simulink model "mod2_2bit_NO_DEM"  (Simulink 7.9)
settings: Solver=ode45  StartTime=0.0  StopTime=simu.trantime  RelTol=1e-3
undefined symbols (not defined in the file): dac, Fs, mod, OSR, sinamp, sinfreq
libraries: simulink x4, dspsigops x3, dsparch4 x1, dspsrcs4 x1
settings Model: Creator=amyles  LastModifiedBy=Arnaldi Isacco
settings DataIOCC: MaxDataPoints=50000  SaveOutput=off  SaveTime=off
settings DebuggingCC: ParameterPrecisionLossMsg=none  StrictBusMsg=Warning
settings SFSimCC: SimParseCustomCode=off
settings CodeAppCC: CustomSymbolStrType=$N$R$M_T
settings GRTTargetCC: CombineOutputUpdateFcns=off  GRTInterface=on

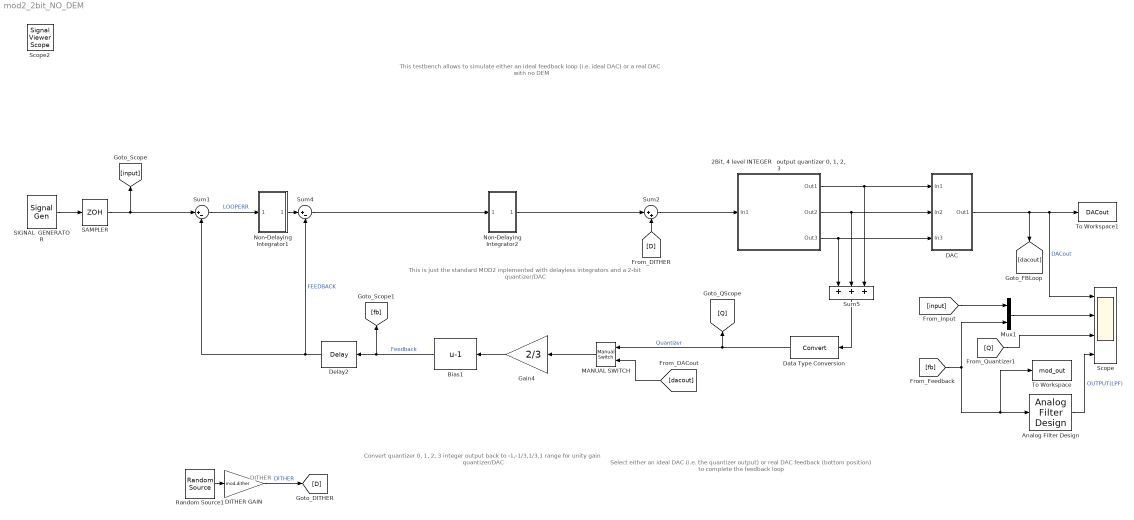
== system mod2_2bit_NO_DEM ==
  note: Convert quantizer 0, 1, 2, 3 integer
      | output back  to -1,-1/3,1/3,1 range for
      | unity gain quantizer/DAC
  note: Select either an ideal DAC
      | (i.e. the quantizer output) or real
      | DAC feedback (bottom position) to
      | complete the feedback loop
  note: This testbench allows to simulate either an ideal feedback loop (i.e. ideal DAC) or a real DAC with no DEM
  note: This is just the standard MOD2 inplemented with delayless integrators and a 2-bit quantizer/DAC
  note: DITHER
  "2Bit, 4 level INTEGER   output quantizer 0, 1, 2, 3" : Subsystem
  Analog Filter Design : dsparch4/Analog Filter Design  method=Butterworth  filttype=Lowpass  N=8  Wlo=pi*(Fs/OSR)  Whi=80  Rp=2  Rs=40
      settings: AttributesFormatString=Low-pass filter the loop output\nto illustrate intuitively how the\npulse density modulated +1/-1\noutput stream does indeed capture\nthe input signal
  Bias1 : Bias  Bias=-1
  DAC : Subsystem
  DITHER GAIN : Gain  Gain=mod.dither  SampleTime=1/Fs
  Data Type Conversion : DataTypeConversion
  Delay2 : dspsigops/Delay  InputProcessing=Columns as channels (frame based)  dly_unit=Samples  delay=1  ic_detail=off  dif_ic_for_ch=off  dif_ic_for_dly=off  ic=0  reset_popup=None
  Gain4 : Gain  Gain=2/3  SampleTime=1/Fs
  MANUAL SWITCH : simulink/Signal Routing/Manual Switch  sw=0  action=0  varsize=off
      settings: AttributesFormatString=Double click to\nselect the desired\ninput
  Mux1 : Mux  Inputs=2
  Non-Delaying Integrator1 : Subsystem
  Non-Delaying Integrator2 : Subsystem
  Random Source1 : dspsrcs4/Random Source  SrcType=Uniform  NormMethod=Ziggurat  CltLength=12  MinVal=-1  MaxVal=1  MeanVal=0  VarVal=1  RepMode=Not repeatable  rawSeed=1  IsInherit=off  SampMode=Discrete  SampTime=1/Fs  SampFrame=1  DataType=Double  OutComplex=Real
  SAMPLER : ZeroOrderHold  SampleTime=1/Fs
  SIGNAL  GENERATOR : SignalGenerator  Amplitude=sinamp  Frequency=sinfreq  VectorParams1D=off
  Scope : Scope  NumInputPorts=4
      settings: YMin=-0.2~-1.1~-0.2~-1.1  YMax=3.2~1.1~3.2~1.1
  Sum1 : Sum  Inputs=|+-  SampleTime=1/Fs
      settings: AttributesFormatString=Modulator input\nloop servo error (input - fbk)
  Sum2 : Sum  Inputs=|++
  Sum4 : Sum  Inputs=|+-
  Sum5 : Sum  Inputs=+++  SampleTime=1/Fs
  To Workspace : ToWorkspace  VariableName=mod_out  SampleTime=-1
  To Workspace1 : ToWorkspace  VariableName=DACout  SampleTime=-1
  Scope2 : SignalViewerScope  IOType=viewer  NumInputPorts=5  ZoomMode=yonly  RefreshTime=0.035000
      settings: YMin=-5~-5~-5~-5~-5  YMax=5~5~5~5~5
  wires:
  Sum1/1 -> Non-Delaying Integrator1/1(In1)  "LOOPERR"
  Delay2/1 -> Sum1/2, Sum4/2  "FEEDBACK"
  SAMPLER/1 -> Sum1/1, [input]
  Sum4/1 -> Non-Delaying Integrator2/1(In1)
  [D] -> Sum2/2
  MANUAL SWITCH/1 -> Gain4/1
  Bias1/1 -> Delay2/1, [fb]  "Feedback"
  Gain4/1 -> Bias1/1
  Sum2/1 -> "2Bit, 4 level INTEGER   output quantizer 0, 1, 2, 3"/1(In1)
  Non-Delaying Integrator1/1(Out1) -> Sum4/1
  Non-Delaying Integrator2/1(Out1) -> Sum2/1
  Data Type Conversion/1 -> MANUAL SWITCH/1, [Q]  "Quantizer"
  [dacout] -> MANUAL SWITCH/2
  "2Bit, 4 level INTEGER   output quantizer 0, 1, 2, 3"/3(Out3) -> Sum5/1, DAC/3(In3)
  "2Bit, 4 level INTEGER   output quantizer 0, 1, 2, 3"/2(Out2) -> Sum5/2, DAC/2(In2)
  Sum5/1 -> Data Type Conversion/1
  "2Bit, 4 level INTEGER   output quantizer 0, 1, 2, 3"/1(Out1) -> Sum5/3, DAC/1(In1)
  DAC/1(Out1) -> [dacout], To Workspace1/1, Scope/1  "DACout"
  [input] -> Mux1/1
  Random Source1/1 -> DITHER GAIN/1
  DITHER GAIN/1 -> [D]  "DITHER"
  SIGNAL  GENERATOR/1 -> SAMPLER/1
  [fb] -> Mux1/2, Analog Filter Design/1, To Workspace/1
  Mux1/1 -> Scope/2
  [Q] -> Scope/3
  Analog Filter Design/1 -> Scope/4  "OUTPUT(LPF)"

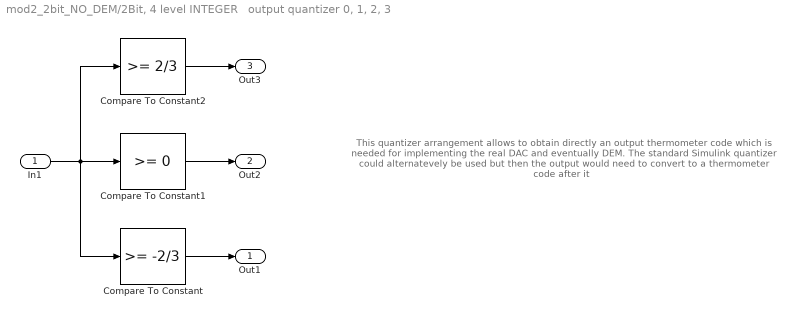
== system mod2_2bit_NO_DEM/2Bit, 4 level INTEGER   output quantizer 0, 1, 2, 3 ==
  note: This quantizer arrangement allows to obtain directly
      | an output thermometer code which is needed for implementing
      | the real DAC and eventually DEM. The standard Simulink
      | quantizer could alternatevely be used but then the output
      | would need to convert to a thermometer code after it
  In1 : Inport
  Compare To Constant : simulink/Logic and Bit Operations/Compare To Constant  relop=>=  const=-2/3  OutDataTypeStr=uint8
  Compare To Constant1 : simulink/Logic and Bit Operations/Compare To Constant  relop=>=  const=0  OutDataTypeStr=uint8
  Compare To Constant2 : simulink/Logic and Bit Operations/Compare To Constant  relop=>=  const=2/3  OutDataTypeStr=uint8
  Out1 : Outport
  Out2 : Outport  Port=2
  Out3 : Outport  Port=3
  wires:
  In1/1 -> Compare To Constant/1, Compare To Constant1/1, Compare To Constant2/1
  Compare To Constant/1 -> Out1/1
  Compare To Constant1/1 -> Out2/1
  Compare To Constant2/1 -> Out3/1

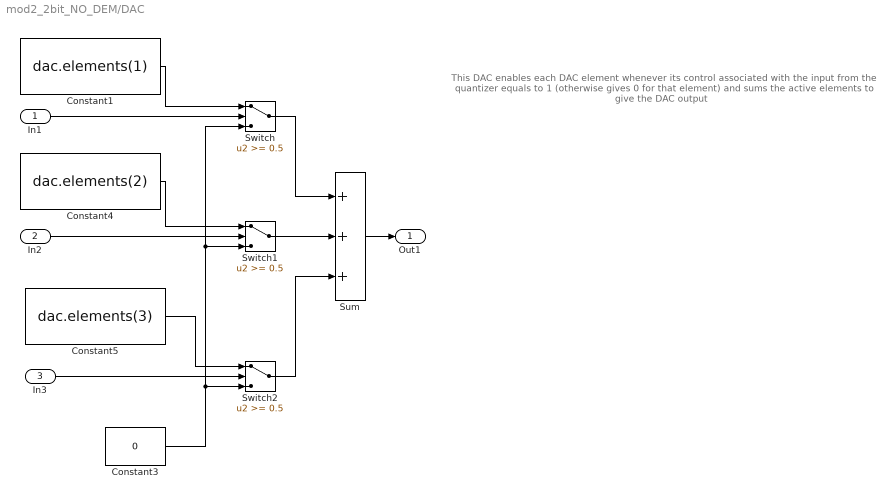
== system mod2_2bit_NO_DEM/DAC ==
  note: This DAC enables each DAC element whenever its control associated
      | with the input from the quantizer equals to 1 (otherwise gives 0 for that
      | element) and sums the active elements to give the DAC output
  In1 : Inport
  In2 : Inport  Port=2
  In3 : Inport  Port=3
  Constant1 : Constant  Value=dac.elements(1)  SampleTime=1/Fs
  Constant3 : Constant  Value=0  SampleTime=1/Fs
  Constant4 : Constant  Value=dac.elements(2)  SampleTime=1/Fs
  Constant5 : Constant  Value=dac.elements(3)  SampleTime=1/Fs
  Sum : Sum  Inputs=+++
  Switch : Switch  Threshold=0.5  SampleTime=1/Fs
  Switch1 : Switch  Threshold=0.5  SampleTime=1/Fs
  Switch2 : Switch  Threshold=0.5  SampleTime=1/Fs
  Out1 : Outport
  wires:
  Switch/1 -> Sum/1
  Switch1/1 -> Sum/2
  Switch2/1 -> Sum/3
  Sum/1 -> Out1/1
  In1/1 -> Switch/2
  In2/1 -> Switch1/2
  In3/1 -> Switch2/2
  Constant1/1 -> Switch/1
  Constant3/1 -> Switch2/3, Switch1/3, Switch/3
  Constant4/1 -> Switch1/1
  Constant5/1 -> Switch2/1

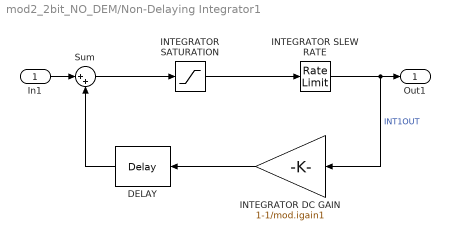
== system mod2_2bit_NO_DEM/Non-Delaying Integrator1 ==
  In1 : Inport
  DELAY : dspsigops/Delay  InputProcessing=Inherited (this choice will be removed - see release notes)  dly_unit=Samples  delay=1  ic_detail=off  dif_ic_for_ch=off  dif_ic_for_dly=off  ic=0  reset_popup=None
  INTEGRATOR SATURATION : Saturate  UpperLimit=mod.isat1  LowerLimit=-(mod.isat1)
      settings: AttributesFormatString=Real integrators will have\noutput swing limits (analog\nsignal headroom or digital\naccumulator min/max values)
  INTEGRATOR SLEW RATE : RateLimiter  RisingSlewLimit=mod.isr1  FallingSlewLimit=-(mod.isr1)  SampleTimeMode=inherited
      settings: AttributesFormatString=...and\nmay suffer from\npoor slew rate
  INTEGRATOR DC GAIN : Gain  Gain=1-1/mod.igain1
      settings: AttributesFormatString=Integrator leakage\n(model finite integrator dc/LF\ngain in analog modulators)
  Sum : Sum  Inputs=|++
      settings: AttributesFormatString=Integrator\nsummer
  Out1 : Outport
  wires:
  DELAY/1 -> Sum/2
  Sum/1 -> INTEGRATOR SATURATION/1
  INTEGRATOR DC GAIN/1 -> DELAY/1
  INTEGRATOR SLEW RATE/1 -> INTEGRATOR DC GAIN/1, Out1/1  "INT1OUT"
  INTEGRATOR SATURATION/1 -> INTEGRATOR SLEW RATE/1
  In1/1 -> Sum/1

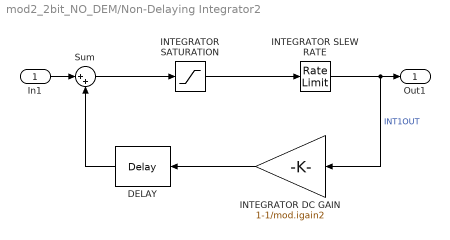
== system mod2_2bit_NO_DEM/Non-Delaying Integrator2 ==
  In1 : Inport
  DELAY : dspsigops/Delay  InputProcessing=Inherited (this choice will be removed - see release notes)  dly_unit=Samples  delay=1  ic_detail=off  dif_ic_for_ch=off  dif_ic_for_dly=off  ic=0  reset_popup=None
  INTEGRATOR SATURATION : Saturate  UpperLimit=mod.isat2  LowerLimit=-(mod.isat2)
      settings: AttributesFormatString=Real integrators will have\noutput swing limits (analog\nsignal headroom or digital\naccumulator min/max values)
  INTEGRATOR SLEW RATE : RateLimiter  RisingSlewLimit=mod.isr2  FallingSlewLimit=-(mod.isr2)  SampleTimeMode=inherited
      settings: AttributesFormatString=...and\nmay suffer from\npoor slew rate
  INTEGRATOR DC GAIN : Gain  Gain=1-1/mod.igain2
      settings: AttributesFormatString=Integrator leakage\n(model finite integrator dc/LF\ngain in analog modulators)
  Sum : Sum  Inputs=|++
      settings: AttributesFormatString=Integrator\nsummer
  Out1 : Outport
  wires:
  DELAY/1 -> Sum/2
  Sum/1 -> INTEGRATOR SATURATION/1
  INTEGRATOR DC GAIN/1 -> DELAY/1
  INTEGRATOR SLEW RATE/1 -> INTEGRATOR DC GAIN/1, Out1/1  "INT1OUT"
  INTEGRATOR SATURATION/1 -> INTEGRATOR SLEW RATE/1
  In1/1 -> Sum/1
